simulink model "heart_model"  (R2015a)
settings: Solver=ode3  StartTime=0.0  StopTime=size(sasignal,1)  FixedStep=1  RelTol=1e-6  AbsTol=1e-6
values from neighbouring files (symbols this model uses):
  beta1 = [-1 -0.3 -0.09 -0.3 -0.3 -0.3 -0.3 -0.3 -0.3 -0.3 -0.3 -0.3 ... (33 elements, 1x33)]    [pacemaker_heart_params.mat]
  beta3 = [200 200 200 200 200 200 200 200 200 200 200 200 ... (33 elements, 1x33)]    [pacemaker_heart_params.mat]
  beta4 = [-0.05 -0.05 -0.02 -0.02 -0.02 -0.02 -0.02 -0.02 -0.02 -0.02 -0.02 -0.02 ... (33 elements, 1x33)]    [pacemaker_heart_params.mat]
  delay = [15.5648 23.2106666667 5.18826666667 12.0149333333 12.8341333333 10.9226666667 18.5685333333 9.55733333333 12.8341333333 4.36906666667 5.46133333333 9.8304 ... (34 elements, 1x34)]    [pacemaker_heart_params.mat]
  gain = [0.1 0.1 0.1 0.1 0.07 0.1 0.1 0.1 0.1 0.1 0.1 0.1 ... (33 elements, 1x33)]    [pacemaker_heart_params.mat]
libraries: simulink x40, dspsrcs4 x1
(part 3 of 5)

== system heart_model/Heart Model/VENTRICLE/RBB (12)/Subsystem3 ==
  q : Inport
  vreset : Inport  Port=2
  reset : Inport  Port=3
  I_st : Inport  Port=4
  vno : Inport  Port=5
  vin : Inport  Port=6
  win : Inport  Port=7
  Constant1 : Constant  Value=0
  Constant2 : Constant  Value=1/6
  Constant3 : Constant
  Gain1 : Gain  Gain=13
  IC : InitialCondition  Value=0
  Integrator : Integrator  ExternalReset=either  InitialConditionSource=external  LimitOutput=on  UpperSaturationLimit=138  ShowStatePort=on
  Math Function : Math  Operator=pow  SaturateOnIntegerOverflow=on
  Subsystem : Subsystem
  Subsystem2 : Subsystem
  Sum : Sum  Inputs=|++
  Switch : Switch  Threshold=0.1
  v : Outport
  vnext : Outport  Port=2
  wires:
  win/1 -> Subsystem/5(win)
  vin/1 -> Subsystem/4(vin), Subsystem2/4(vin)
  Integrator/State -> vnext/1
  Constant1/1 -> Switch/3
  vno/1 -> Switch/1, Switch/2
  Sum/1 -> Subsystem/3(f(vno))
  Switch/1 -> Math Function/1
  Constant3/1 -> Sum/2
  Gain1/1 -> Sum/1
  Math Function/1 -> Gain1/1
  Constant2/1 -> Math Function/2
  I_st/1 -> Subsystem2/1(I_st)
  reset/1 -> Integrator/2
  vreset/1 -> IC/1
  Subsystem2/1(vint) -> Integrator/1
  Subsystem/1(vgain) -> Subsystem2/3(vgain)
  Integrator/1 -> Subsystem/2(v), v/1
  IC/1 -> Integrator/3
  q/1 -> Subsystem/1(q), Subsystem2/2(q)

== system heart_model/Heart Model/VENTRICLE/RBB_m (11)/Subsystem3 ==
  q : Inport
  vreset : Inport  Port=2
  reset : Inport  Port=3
  I_st : Inport  Port=4
  vno : Inport  Port=5
  vin : Inport  Port=6
  win : Inport  Port=7
  Constant1 : Constant  Value=0
  Constant2 : Constant  Value=1/6
  Constant3 : Constant
  Gain1 : Gain  Gain=13
  IC : InitialCondition  Value=0
  Integrator : Integrator  ExternalReset=either  InitialConditionSource=external  LimitOutput=on  UpperSaturationLimit=138  ShowStatePort=on
  Math Function : Math  Operator=pow  SaturateOnIntegerOverflow=on
  Subsystem : Subsystem
  Subsystem2 : Subsystem
  Sum : Sum  Inputs=|++
  Switch : Switch  Threshold=0.1
  v : Outport
  vnext : Outport  Port=2
  wires:
  win/1 -> Subsystem/5(win)
  vin/1 -> Subsystem/4(vin), Subsystem2/4(vin)
  Integrator/State -> vnext/1
  Constant1/1 -> Switch/3
  vno/1 -> Switch/1, Switch/2
  Sum/1 -> Subsystem/3(f(vno))
  Switch/1 -> Math Function/1
  Constant3/1 -> Sum/2
  Gain1/1 -> Sum/1
  Math Function/1 -> Gain1/1
  Constant2/1 -> Math Function/2
  I_st/1 -> Subsystem2/1(I_st)
  reset/1 -> Integrator/2
  vreset/1 -> IC/1
  Subsystem2/1(vint) -> Integrator/1
  Subsystem/1(vgain) -> Subsystem2/3(vgain)
  Integrator/1 -> Subsystem/2(v), v/1
  IC/1 -> Integrator/3
  q/1 -> Subsystem/1(q), Subsystem2/2(q)

== system heart_model/Heart Model/VENTRICLE/RV (18)/Subsystem3 ==
  q : Inport
  vreset : Inport  Port=2
  reset : Inport  Port=3
  I_st : Inport  Port=4
  vno : Inport  Port=5
  vin : Inport  Port=6
  win : Inport  Port=7
  Constant1 : Constant  Value=0
  Constant2 : Constant  Value=1/6
  Constant3 : Constant
  Gain1 : Gain  Gain=13
  IC : InitialCondition  Value=0
  Integrator : Integrator  ExternalReset=either  InitialConditionSource=external  LimitOutput=on  UpperSaturationLimit=138  ShowStatePort=on
  Math Function : Math  Operator=pow  SaturateOnIntegerOverflow=on
  Subsystem : Subsystem
  Subsystem2 : Subsystem
  Sum : Sum  Inputs=|++
  Switch : Switch  Threshold=0.1
  v : Outport
  vnext : Outport  Port=2
  wires:
  win/1 -> Subsystem/5(win)
  vin/1 -> Subsystem/4(vin), Subsystem2/4(vin)
  Integrator/State -> vnext/1
  Constant1/1 -> Switch/3
  vno/1 -> Switch/1, Switch/2
  Sum/1 -> Subsystem/3(f(vno))
  Switch/1 -> Math Function/1
  Constant3/1 -> Sum/2
  Gain1/1 -> Sum/1
  Math Function/1 -> Gain1/1
  Constant2/1 -> Math Function/2
  I_st/1 -> Subsystem2/1(I_st)
  reset/1 -> Integrator/2
  vreset/1 -> IC/1
  Subsystem2/1(vint) -> Integrator/1
  Subsystem/1(vgain) -> Subsystem2/3(vgain)
  Integrator/1 -> Subsystem/2(v), v/1
  IC/1 -> Integrator/3
  q/1 -> Subsystem/1(q), Subsystem2/2(q)

== system heart_model/Heart Model/VENTRICLE/RVA (15)/Subsystem3 ==
  q : Inport
  vreset : Inport  Port=2
  reset : Inport  Port=3
  I_st : Inport  Port=4
  vno : Inport  Port=5
  vin : Inport  Port=6
  win : Inport  Port=7
  Constant1 : Constant  Value=0
  Constant2 : Constant  Value=1/6
  Constant3 : Constant
  Gain1 : Gain  Gain=13
  IC : InitialCondition  Value=0
  Integrator : Integrator  ExternalReset=either  InitialConditionSource=external  LimitOutput=on  UpperSaturationLimit=138  ShowStatePort=on
  Math Function : Math  Operator=pow  SaturateOnIntegerOverflow=on
  Subsystem : Subsystem
  Subsystem2 : Subsystem
  Sum : Sum  Inputs=|++
  Switch : Switch  Threshold=0.1
  v : Outport
  vnext : Outport  Port=2
  wires:
  win/1 -> Subsystem/5(win)
  vin/1 -> Subsystem/4(vin), Subsystem2/4(vin)
  Integrator/State -> vnext/1
  Constant1/1 -> Switch/3
  vno/1 -> Switch/1, Switch/2
  Sum/1 -> Subsystem/3(f(vno))
  Switch/1 -> Math Function/1
  Constant3/1 -> Sum/2
  Gain1/1 -> Sum/1
  Math Function/1 -> Gain1/1
  Constant2/1 -> Math Function/2
  I_st/1 -> Subsystem2/1(I_st)
  reset/1 -> Integrator/2
  vreset/1 -> IC/1
  Subsystem2/1(vint) -> Integrator/1
  Subsystem/1(vgain) -> Subsystem2/3(vgain)
  Integrator/1 -> Subsystem/2(v), v/1
  IC/1 -> Integrator/3
  q/1 -> Subsystem/1(q), Subsystem2/2(q)

== system heart_model/Heart Model/VENTRICLE/RV_m (17)/Subsystem3 ==
  q : Inport
  vreset : Inport  Port=2
  reset : Inport  Port=3
  I_st : Inport  Port=4
  vno : Inport  Port=5
  vin : Inport  Port=6
  win : Inport  Port=7
  Constant1 : Constant  Value=0
  Constant2 : Constant  Value=1/6
  Constant3 : Constant
  Gain1 : Gain  Gain=13
  IC : InitialCondition  Value=0
  Integrator : Integrator  ExternalReset=either  InitialConditionSource=external  LimitOutput=on  UpperSaturationLimit=138  ShowStatePort=on
  Math Function : Math  Operator=pow  SaturateOnIntegerOverflow=on
  Subsystem : Subsystem
  Subsystem2 : Subsystem
  Sum : Sum  Inputs=|++
  Switch : Switch  Threshold=0.1
  v : Outport
  vnext : Outport  Port=2
  wires:
  win/1 -> Subsystem/5(win)
  vin/1 -> Subsystem/4(vin), Subsystem2/4(vin)
  Integrator/State -> vnext/1
  Constant1/1 -> Switch/3
  vno/1 -> Switch/1, Switch/2
  Sum/1 -> Subsystem/3(f(vno))
  Switch/1 -> Math Function/1
  Constant3/1 -> Sum/2
  Gain1/1 -> Sum/1
  Math Function/1 -> Gain1/1
  Constant2/1 -> Math Function/2
  I_st/1 -> Subsystem2/1(I_st)
  reset/1 -> Integrator/2
  vreset/1 -> IC/1
  Subsystem2/1(vint) -> Integrator/1
  Subsystem/1(vgain) -> Subsystem2/3(vgain)
  Integrator/1 -> Subsystem/2(v), v/1
  IC/1 -> Integrator/3
  q/1 -> Subsystem/1(q), Subsystem2/2(q)

== system heart_model/Heart Model/VENTRICLE/SEP_LV (27)/Subsystem3 ==
  q : Inport
  vreset : Inport  Port=2
  reset : Inport  Port=3
  I_st : Inport  Port=4
  vno : Inport  Port=5
  vin : Inport  Port=6
  win : Inport  Port=7
  Constant1 : Constant  Value=0
  Constant2 : Constant  Value=1/6
  Constant3 : Constant
  Gain1 : Gain  Gain=13
  IC : InitialCondition  Value=0
  Integrator : Integrator  ExternalReset=either  InitialConditionSource=external  LimitOutput=on  UpperSaturationLimit=138  ShowStatePort=on
  Math Function : Math  Operator=pow  SaturateOnIntegerOverflow=on
  Subsystem : Subsystem
  Subsystem2 : Subsystem
  Sum : Sum  Inputs=|++
  Switch : Switch  Threshold=0.1
  v : Outport
  vnext : Outport  Port=2
  wires:
  win/1 -> Subsystem/5(win)
  vin/1 -> Subsystem/4(vin), Subsystem2/4(vin)
  Integrator/State -> vnext/1
  Constant1/1 -> Switch/3
  vno/1 -> Switch/1, Switch/2
  Sum/1 -> Subsystem/3(f(vno))
  Switch/1 -> Math Function/1
  Constant3/1 -> Sum/2
  Gain1/1 -> Sum/1
  Math Function/1 -> Gain1/1
  Constant2/1 -> Math Function/2
  I_st/1 -> Subsystem2/1(I_st)
  reset/1 -> Integrator/2
  vreset/1 -> IC/1
  Subsystem2/1(vint) -> Integrator/1
  Subsystem/1(vgain) -> Subsystem2/3(vgain)
  Integrator/1 -> Subsystem/2(v), v/1
  IC/1 -> Integrator/3
  q/1 -> Subsystem/1(q), Subsystem2/2(q)

== system heart_model/Heart Model/VENTRICLE/SEP_LV_m (26)/Subsystem3 ==
  q : Inport
  vreset : Inport  Port=2
  reset : Inport  Port=3
  I_st : Inport  Port=4
  vno : Inport  Port=5
  vin : Inport  Port=6
  win : Inport  Port=7
  Constant1 : Constant  Value=0
  Constant2 : Constant  Value=1/6
  Constant3 : Constant
  Gain1 : Gain  Gain=13
  IC : InitialCondition  Value=0
  Integrator : Integrator  ExternalReset=either  InitialConditionSource=external  LimitOutput=on  UpperSaturationLimit=138  ShowStatePort=on
  Math Function : Math  Operator=pow  SaturateOnIntegerOverflow=on
  Subsystem : Subsystem
  Subsystem2 : Subsystem
  Sum : Sum  Inputs=|++
  Switch : Switch  Threshold=0.1
  v : Outport
  vnext : Outport  Port=2
  wires:
  win/1 -> Subsystem/5(win)
  vin/1 -> Subsystem/4(vin), Subsystem2/4(vin)
  Integrator/State -> vnext/1
  Constant1/1 -> Switch/3
  vno/1 -> Switch/1, Switch/2
  Sum/1 -> Subsystem/3(f(vno))
  Switch/1 -> Math Function/1
  Constant3/1 -> Sum/2
  Gain1/1 -> Sum/1
  Math Function/1 -> Gain1/1
  Constant2/1 -> Math Function/2
  I_st/1 -> Subsystem2/1(I_st)
  reset/1 -> Integrator/2
  vreset/1 -> IC/1
  Subsystem2/1(vint) -> Integrator/1
  Subsystem/1(vgain) -> Subsystem2/3(vgain)
  Integrator/1 -> Subsystem/2(v), v/1
  IC/1 -> Integrator/3
  q/1 -> Subsystem/1(q), Subsystem2/2(q)

== system heart_model/Heart Model/VENTRICLE/SEP_RV (25)/Subsystem3 ==
  q : Inport
  vreset : Inport  Port=2
  reset : Inport  Port=3
  I_st : Inport  Port=4
  vno : Inport  Port=5
  vin : Inport  Port=6
  win : Inport  Port=7
  Constant1 : Constant  Value=0
  Constant2 : Constant  Value=1/6
  Constant3 : Constant
  Gain1 : Gain  Gain=13
  IC : InitialCondition  Value=0
  Integrator : Integrator  ExternalReset=either  InitialConditionSource=external  LimitOutput=on  UpperSaturationLimit=138  ShowStatePort=on
  Math Function : Math  Operator=pow  SaturateOnIntegerOverflow=on
  Subsystem : Subsystem
  Subsystem2 : Subsystem
  Sum : Sum  Inputs=|++
  Switch : Switch  Threshold=0.1
  v : Outport
  vnext : Outport  Port=2
  wires:
  win/1 -> Subsystem/5(win)
  vin/1 -> Subsystem/4(vin), Subsystem2/4(vin)
  Integrator/State -> vnext/1
  Constant1/1 -> Switch/3
  vno/1 -> Switch/1, Switch/2
  Sum/1 -> Subsystem/3(f(vno))
  Switch/1 -> Math Function/1
  Constant3/1 -> Sum/2
  Gain1/1 -> Sum/1
  Math Function/1 -> Gain1/1
  Constant2/1 -> Math Function/2
  I_st/1 -> Subsystem2/1(I_st)
  reset/1 -> Integrator/2
  vreset/1 -> IC/1
  Subsystem2/1(vint) -> Integrator/1
  Subsystem/1(vgain) -> Subsystem2/3(vgain)
  Integrator/1 -> Subsystem/2(v), v/1
  IC/1 -> Integrator/3
  q/1 -> Subsystem/1(q), Subsystem2/2(q)

== system heart_model/Heart Model/VENTRICLE/SEP_RV_m (24)/Subsystem3 ==
  q : Inport
  vreset : Inport  Port=2
  reset : Inport  Port=3
  I_st : Inport  Port=4
  vno : Inport  Port=5
  vin : Inport  Port=6
  win : Inport  Port=7
  Constant1 : Constant  Value=0
  Constant2 : Constant  Value=1/6
  Constant3 : Constant
  Gain1 : Gain  Gain=13
  IC : InitialCondition  Value=0
  Integrator : Integrator  ExternalReset=either  InitialConditionSource=external  LimitOutput=on  UpperSaturationLimit=138  ShowStatePort=on
  Math Function : Math  Operator=pow  SaturateOnIntegerOverflow=on
  Subsystem : Subsystem
  Subsystem2 : Subsystem
  Sum : Sum  Inputs=|++
  Switch : Switch  Threshold=0.1
  v : Outport
  vnext : Outport  Port=2
  wires:
  win/1 -> Subsystem/5(win)
  vin/1 -> Subsystem/4(vin), Subsystem2/4(vin)
  Integrator/State -> vnext/1
  Constant1/1 -> Switch/3
  vno/1 -> Switch/1, Switch/2
  Sum/1 -> Subsystem/3(f(vno))
  Switch/1 -> Math Function/1
  Constant3/1 -> Sum/2
  Gain1/1 -> Sum/1
  Math Function/1 -> Gain1/1
  Constant2/1 -> Math Function/2
  I_st/1 -> Subsystem2/1(I_st)
  reset/1 -> Integrator/2
  vreset/1 -> IC/1
  Subsystem2/1(vint) -> Integrator/1
  Subsystem/1(vgain) -> Subsystem2/3(vgain)
  Integrator/1 -> Subsystem/2(v), v/1
  IC/1 -> Integrator/3
  q/1 -> Subsystem/1(q), Subsystem2/2(q)

== system heart_model/Heart Model/ATRIUM/Bach (8)/Subsystem3/Subsystem ==
  q : Inport
  v : Inport  Port=2
  f(vno) : Inport  Port=3
  vin : Inport  Port=4
  win : Inport  Port=5
  Gain3 : Gain  Gain=-1
  Multiport Switch : MultiPortSwitch  Inputs=4
  Product : Product  RndMeth=Zero
  Product1 : Product  RndMeth=Zero
  Sum : Sum  Inputs=|++
  Sum1 : Sum  Inputs=|++
  beta1 : Gain  Gain=beta1(8)
  beta3 : Gain  Gain=beta3(8)
  beta4 : Gain  Gain=beta4(8)
  vgain : Outport
  wires:
  Gain3/1 -> Product1/2
  Product1/1 -> Multiport Switch/3, Sum1/2
  Sum1/1 -> Multiport Switch/2
  Sum/1 -> Sum1/1
  win/1 -> Gain3/1
  vin/1 -> Sum/1
  beta1/1 -> Sum/2
  f(vno)/1 -> Product/2
  beta4/1 -> Product/1
  Product/1 -> Multiport Switch/5
  v/1 -> Product1/1, beta4/1, beta3/1, beta1/1
  beta3/1 -> Multiport Switch/4
  Multiport Switch/1 -> vgain/1
  q/1 -> Multiport Switch/1

== system heart_model/Heart Model/ATRIUM/Bach (8)/Subsystem3/Subsystem2 ==
  I_st : Inport
  q : Inport  Port=2
  vgain : Inport  Port=3
  vin : Inport  Port=4
  Compare To Constant : simulink/Logic and Bit Operations/Compare To Constant  relop===  const=2  OutDataTypeStr=uint8
  Sum : Sum  Inputs=|++
  Sum1 : Sum  Inputs=|++
  Switch : Switch  Criteria=u2 ~= 0
  vint : Outport
  wires:
  Sum1/1 -> Switch/1
  Sum/1 -> Sum1/2
  vin/1 -> Sum/2
  I_st/1 -> Sum/1
  vgain/1 -> Sum1/1, Switch/3
  Switch/1 -> vint/1
  q/1 -> Compare To Constant/1
  Compare To Constant/1 -> Switch/2

== system heart_model/Heart Model/ATRIUM/CS_LA (29)/Subsystem3/Subsystem ==
  q : Inport
  v : Inport  Port=2
  f(vno) : Inport  Port=3
  vin : Inport  Port=4
  win : Inport  Port=5
  Gain3 : Gain  Gain=-1
  Multiport Switch : MultiPortSwitch  Inputs=4
  Product : Product  RndMeth=Zero
  Product1 : Product  RndMeth=Zero
  Sum : Sum  Inputs=|++
  Sum1 : Sum  Inputs=|++
  beta1 : Gain  Gain=beta1(29)
  beta3 : Gain  Gain=beta3(29)
  beta4 : Gain  Gain=beta4(29)
  vgain : Outport
  wires:
  Gain3/1 -> Product1/2
  Product1/1 -> Multiport Switch/3, Sum1/2
  Sum1/1 -> Multiport Switch/2
  Sum/1 -> Sum1/1
  win/1 -> Gain3/1
  vin/1 -> Sum/1
  beta1/1 -> Sum/2
  f(vno)/1 -> Product/2
  beta4/1 -> Product/1
  Product/1 -> Multiport Switch/5
  v/1 -> Product1/1, beta4/1, beta3/1, beta1/1
  beta3/1 -> Multiport Switch/4
  Multiport Switch/1 -> vgain/1
  q/1 -> Multiport Switch/1

== system heart_model/Heart Model/ATRIUM/CS_LA (29)/Subsystem3/Subsystem2 ==
  I_st : Inport
  q : Inport  Port=2
  vgain : Inport  Port=3
  vin : Inport  Port=4
  Compare To Constant : simulink/Logic and Bit Operations/Compare To Constant  relop===  const=2  OutDataTypeStr=uint8
  Sum : Sum  Inputs=|++
  Sum1 : Sum  Inputs=|++
  Switch : Switch  Criteria=u2 ~= 0
  vint : Outport
  wires:
  Sum1/1 -> Switch/1
  Sum/1 -> Sum1/2
  vin/1 -> Sum/2
  I_st/1 -> Sum/1
  vgain/1 -> Sum1/1, Switch/3
  Switch/1 -> vint/1
  q/1 -> Compare To Constant/1
  Compare To Constant/1 -> Switch/2

== system heart_model/Heart Model/ATRIUM/CT (2)/Subsystem3/Subsystem ==
  q : Inport
  v : Inport  Port=2
  f(vno) : Inport  Port=3
  vin : Inport  Port=4
  win : Inport  Port=5
  Gain3 : Gain  Gain=-1
  Multiport Switch : MultiPortSwitch  Inputs=4
  Product : Product  RndMeth=Zero
  Product1 : Product  RndMeth=Zero
  Sum : Sum  Inputs=|++
  Sum1 : Sum  Inputs=|++
  beta1 : Gain  Gain=beta1(2)
  beta3 : Gain  Gain=beta3(2)
  beta4 : Gain  Gain=beta4(2)
  vgain : Outport
  wires:
  Gain3/1 -> Product1/2
  Product1/1 -> Multiport Switch/3, Sum1/2
  Sum1/1 -> Multiport Switch/2
  Sum/1 -> Sum1/1
  win/1 -> Gain3/1
  vin/1 -> Sum/1
  beta1/1 -> Sum/2
  f(vno)/1 -> Product/2
  beta4/1 -> Product/1
  Product/1 -> Multiport Switch/5
  v/1 -> Product1/1, beta4/1, beta3/1, beta1/1
  beta3/1 -> Multiport Switch/4
  Multiport Switch/1 -> vgain/1
  q/1 -> Multiport Switch/1

== system heart_model/Heart Model/ATRIUM/CT (2)/Subsystem3/Subsystem2 ==
  I_st : Inport
  q : Inport  Port=2
  vgain : Inport  Port=3
  vin : Inport  Port=4
  Compare To Constant : simulink/Logic and Bit Operations/Compare To Constant  relop===  const=2  OutDataTypeStr=uint8
  Sum : Sum  Inputs=|++
  Sum1 : Sum  Inputs=|++
  Switch : Switch  Criteria=u2 ~= 0
  vint : Outport
  wires:
  Sum1/1 -> Switch/1
  Sum/1 -> Sum1/2
  vin/1 -> Sum/2
  I_st/1 -> Sum/1
  vgain/1 -> Sum1/1, Switch/3
  Switch/1 -> vint/1
  q/1 -> Compare To Constant/1
  Compare To Constant/1 -> Switch/2

== system heart_model/Heart Model/ATRIUM/CT_a (21)/Subsystem3/Subsystem ==
  q : Inport
  v : Inport  Port=2
  f(vno) : Inport  Port=3
  vin : Inport  Port=4
  win : Inport  Port=5
  Gain3 : Gain  Gain=-1
  Multiport Switch : MultiPortSwitch  Inputs=4
  Product : Product  RndMeth=Zero
  Product1 : Product  RndMeth=Zero
  Sum : Sum  Inputs=|++
  Sum1 : Sum  Inputs=|++
  beta1 : Gain  Gain=beta1(21)
  beta3 : Gain  Gain=beta3(21)
  beta4 : Gain  Gain=beta4(21)
  vgain : Outport
  wires:
  Gain3/1 -> Product1/2
  Product1/1 -> Multiport Switch/3, Sum1/2
  Sum1/1 -> Multiport Switch/2
  Sum/1 -> Sum1/1
  win/1 -> Gain3/1
  vin/1 -> Sum/1
  beta1/1 -> Sum/2
  f(vno)/1 -> Product/2
  beta4/1 -> Product/1
  Product/1 -> Multiport Switch/5
  v/1 -> Product1/1, beta4/1, beta3/1, beta1/1
  beta3/1 -> Multiport Switch/4
  Multiport Switch/1 -> vgain/1
  q/1 -> Multiport Switch/1

== system heart_model/Heart Model/ATRIUM/CT_a (21)/Subsystem3/Subsystem2 ==
  I_st : Inport
  q : Inport  Port=2
  vgain : Inport  Port=3
  vin : Inport  Port=4
  Compare To Constant : simulink/Logic and Bit Operations/Compare To Constant  relop===  const=2  OutDataTypeStr=uint8
  Sum : Sum  Inputs=|++
  Sum1 : Sum  Inputs=|++
  Switch : Switch  Criteria=u2 ~= 0
  vint : Outport
  wires:
  Sum1/1 -> Switch/1
  Sum/1 -> Sum1/2
  vin/1 -> Sum/2
  I_st/1 -> Sum/1
  vgain/1 -> Sum1/1, Switch/3
  Switch/1 -> vint/1
  q/1 -> Compare To Constant/1
  Compare To Constant/1 -> Switch/2

== system heart_model/Heart Model/ATRIUM/Fast (32)/Subsystem3/Subsystem ==
  q : Inport
  v : Inport  Port=2
  f(vno) : Inport  Port=3
  vin : Inport  Port=4
  win : Inport  Port=5
  Gain3 : Gain  Gain=-1
  Multiport Switch : MultiPortSwitch  Inputs=4
  Product : Product  RndMeth=Zero
  Product1 : Product  RndMeth=Zero
  Sum : Sum  Inputs=|++
  Sum1 : Sum  Inputs=|++
  beta1 : Gain  Gain=beta1(32)
  beta3 : Gain  Gain=beta3(32)
  beta4 : Gain  Gain=beta4(32)
  vgain : Outport
  wires:
  Gain3/1 -> Product1/2
  Product1/1 -> Multiport Switch/3, Sum1/2
  Sum1/1 -> Multiport Switch/2
  Sum/1 -> Sum1/1
  win/1 -> Gain3/1
  vin/1 -> Sum/1
  beta1/1 -> Sum/2
  f(vno)/1 -> Product/2
  beta4/1 -> Product/1
  Product/1 -> Multiport Switch/5
  v/1 -> Product1/1, beta4/1, beta3/1, beta1/1
  beta3/1 -> Multiport Switch/4
  Multiport Switch/1 -> vgain/1
  q/1 -> Multiport Switch/1

== system heart_model/Heart Model/ATRIUM/Fast (32)/Subsystem3/Subsystem2 ==
  I_st : Inport
  q : Inport  Port=2
  vgain : Inport  Port=3
  vin : Inport  Port=4
  Compare To Constant : simulink/Logic and Bit Operations/Compare To Constant  relop===  const=2  OutDataTypeStr=uint8
  Sum : Sum  Inputs=|++
  Sum1 : Sum  Inputs=|++
  Switch : Switch  Criteria=u2 ~= 0
  vint : Outport
  wires:
  Sum1/1 -> Switch/1
  Sum/1 -> Sum1/2
  vin/1 -> Sum/2
  I_st/1 -> Sum/1
  vgain/1 -> Sum1/1, Switch/3
  Switch/1 -> vint/1
  q/1 -> Compare To Constant/1
  Compare To Constant/1 -> Switch/2

== system heart_model/Heart Model/ATRIUM/Fast_b (33)/Subsystem3/Subsystem ==
  q : Inport
  v : Inport  Port=2
  f(vno) : Inport  Port=3
  vin : Inport  Port=4
  win : Inport  Port=5
  Gain3 : Gain  Gain=-1
  Multiport Switch : MultiPortSwitch  Inputs=4
  Product : Product  RndMeth=Zero
  Product1 : Product  RndMeth=Zero
  Sum : Sum  Inputs=|++
  Sum1 : Sum  Inputs=|++
  beta1 : Gain  Gain=beta1(33)
  beta3 : Gain  Gain=beta3(33)
  beta4 : Gain  Gain=beta4(33)
  vgain : Outport
  wires:
  Gain3/1 -> Product1/2
  Product1/1 -> Multiport Switch/3, Sum1/2
  Sum1/1 -> Multiport Switch/2
  Sum/1 -> Sum1/1
  win/1 -> Gain3/1
  vin/1 -> Sum/1
  beta1/1 -> Sum/2
  f(vno)/1 -> Product/2
  beta4/1 -> Product/1
  Product/1 -> Multiport Switch/5
  v/1 -> Product1/1, beta4/1, beta3/1, beta1/1
  beta3/1 -> Multiport Switch/4
  Multiport Switch/1 -> vgain/1
  q/1 -> Multiport Switch/1

== system heart_model/Heart Model/ATRIUM/Fast_b (33)/Subsystem3/Subsystem2 ==
  I_st : Inport
  q : Inport  Port=2
  vgain : Inport  Port=3
  vin : Inport  Port=4
  Compare To Constant : simulink/Logic and Bit Operations/Compare To Constant  relop===  const=2  OutDataTypeStr=uint8
  Sum : Sum  Inputs=|++
  Sum1 : Sum  Inputs=|++
  Switch : Switch  Criteria=u2 ~= 0
  vint : Outport
  wires:
  Sum1/1 -> Switch/1
  Sum/1 -> Sum1/2
  vin/1 -> Sum/2
  I_st/1 -> Sum/1
  vgain/1 -> Sum1/1, Switch/3
  Switch/1 -> vint/1
  q/1 -> Compare To Constant/1
  Compare To Constant/1 -> Switch/2

== system heart_model/Heart Model/ATRIUM/LA (10)/Subsystem3/Subsystem ==
  q : Inport
  v : Inport  Port=2
  f(vno) : Inport  Port=3
  vin : Inport  Port=4
  win : Inport  Port=5
  Gain3 : Gain  Gain=-1
  Multiport Switch : MultiPortSwitch  Inputs=4
  Product : Product  RndMeth=Zero
  Product1 : Product  RndMeth=Zero
  Sum : Sum  Inputs=|++
  Sum1 : Sum  Inputs=|++
  beta1 : Gain  Gain=beta1(10)
  beta3 : Gain  Gain=beta3(10)
  beta4 : Gain  Gain=beta4(10)
  vgain : Outport
  wires:
  Gain3/1 -> Product1/2
  Product1/1 -> Multiport Switch/3, Sum1/2
  Sum1/1 -> Multiport Switch/2
  Sum/1 -> Sum1/1
  win/1 -> Gain3/1
  vin/1 -> Sum/1
  beta1/1 -> Sum/2
  f(vno)/1 -> Product/2
  beta4/1 -> Product/1
  Product/1 -> Multiport Switch/5
  v/1 -> Product1/1, beta4/1, beta3/1, beta1/1
  beta3/1 -> Multiport Switch/4
  Multiport Switch/1 -> vgain/1
  q/1 -> Multiport Switch/1

== system heart_model/Heart Model/ATRIUM/LA (10)/Subsystem3/Subsystem2 ==
  I_st : Inport
  q : Inport  Port=2
  vgain : Inport  Port=3
  vin : Inport  Port=4
  Compare To Constant : simulink/Logic and Bit Operations/Compare To Constant  relop===  const=2  OutDataTypeStr=uint8
  Sum : Sum  Inputs=|++
  Sum1 : Sum  Inputs=|++
  Switch : Switch  Criteria=u2 ~= 0
  vint : Outport
  wires:
  Sum1/1 -> Switch/1
  Sum/1 -> Sum1/2
  vin/1 -> Sum/2
  I_st/1 -> Sum/1
  vgain/1 -> Sum1/1, Switch/3
  Switch/1 -> vint/1
  q/1 -> Compare To Constant/1
  Compare To Constant/1 -> Switch/2

== system heart_model/Heart Model/ATRIUM/LA_a (9)/Subsystem3/Subsystem ==
  q : Inport
  v : Inport  Port=2
  f(vno) : Inport  Port=3
  vin : Inport  Port=4
  win : Inport  Port=5
  Gain3 : Gain  Gain=-1
  Multiport Switch : MultiPortSwitch  Inputs=4
  Product : Product  RndMeth=Zero
  Product1 : Product  RndMeth=Zero
  Sum : Sum  Inputs=|++
  Sum1 : Sum  Inputs=|++
  beta1 : Gain  Gain=beta1(9)
  beta3 : Gain  Gain=beta3(9)
  beta4 : Gain  Gain=beta4(9)
  vgain : Outport
  wires:
  Gain3/1 -> Product1/2
  Product1/1 -> Multiport Switch/3, Sum1/2
  Sum1/1 -> Multiport Switch/2
  Sum/1 -> Sum1/1
  win/1 -> Gain3/1
  vin/1 -> Sum/1
  beta1/1 -> Sum/2
  f(vno)/1 -> Product/2
  beta4/1 -> Product/1
  Product/1 -> Multiport Switch/5
  v/1 -> Product1/1, beta4/1, beta3/1, beta1/1
  beta3/1 -> Multiport Switch/4
  Multiport Switch/1 -> vgain/1
  q/1 -> Multiport Switch/1

== system heart_model/Heart Model/ATRIUM/LA_a (9)/Subsystem3/Subsystem2 ==
  I_st : Inport
  q : Inport  Port=2
  vgain : Inport  Port=3
  vin : Inport  Port=4
  Compare To Constant : simulink/Logic and Bit Operations/Compare To Constant  relop===  const=2  OutDataTypeStr=uint8
  Sum : Sum  Inputs=|++
  Sum1 : Sum  Inputs=|++
  Switch : Switch  Criteria=u2 ~= 0
  vint : Outport
  wires:
  Sum1/1 -> Switch/1
  Sum/1 -> Sum1/2
  vin/1 -> Sum/2
  I_st/1 -> Sum/1
  vgain/1 -> Sum1/1, Switch/3
  Switch/1 -> vint/1
  q/1 -> Compare To Constant/1
  Compare To Constant/1 -> Switch/2

== system heart_model/Heart Model/ATRIUM/OS (4)/Subsystem3/Subsystem ==
  q : Inport
  v : Inport  Port=2
  f(vno) : Inport  Port=3
  vin : Inport  Port=4
  win : Inport  Port=5
  Gain3 : Gain  Gain=-1
  Multiport Switch : MultiPortSwitch  Inputs=4
  Product : Product  RndMeth=Zero
  Product1 : Product  RndMeth=Zero
  Sum : Sum  Inputs=|++
  Sum1 : Sum  Inputs=|++
  beta1 : Gain  Gain=beta1(4)
  beta3 : Gain  Gain=beta3(4)
  beta4 : Gain  Gain=beta4(4)
  vgain : Outport
  wires:
  Gain3/1 -> Product1/2
  Product1/1 -> Multiport Switch/3, Sum1/2
  Sum1/1 -> Multiport Switch/2
  Sum/1 -> Sum1/1
  win/1 -> Gain3/1
  vin/1 -> Sum/1
  beta1/1 -> Sum/2
  f(vno)/1 -> Product/2
  beta4/1 -> Product/1
  Product/1 -> Multiport Switch/5
  v/1 -> Product1/1, beta4/1, beta3/1, beta1/1
  beta3/1 -> Multiport Switch/4
  Multiport Switch/1 -> vgain/1
  q/1 -> Multiport Switch/1

== system heart_model/Heart Model/ATRIUM/OS (4)/Subsystem3/Subsystem2 ==
  I_st : Inport
  q : Inport  Port=2
  vgain : Inport  Port=3
  Compare To Constant : simulink/Logic and Bit Operations/Compare To Constant  relop===  const=2  OutDataTypeStr=uint8
  Switch : Switch  Criteria=u2 ~= 0
  vint : Outport
  wires:
  I_st/1 -> Switch/1
  vgain/1 -> Switch/3
  Switch/1 -> vint/1
  q/1 -> Compare To Constant/1
  Compare To Constant/1 -> Switch/2

== system heart_model/Heart Model/ATRIUM/RA (23)/Subsystem3/Subsystem ==
  q : Inport
  v : Inport  Port=2
  f(vno) : Inport  Port=3
  vin : Inport  Port=4
  win : Inport  Port=5
  Gain3 : Gain  Gain=-1
  Multiport Switch : MultiPortSwitch  Inputs=4
  Product : Product  RndMeth=Zero
  Product1 : Product  RndMeth=Zero
  Sum : Sum  Inputs=|++
  Sum1 : Sum  Inputs=|++
  beta1 : Gain  Gain=beta1(23)
  beta3 : Gain  Gain=beta3(23)
  beta4 : Gain  Gain=beta4(23)
  vgain : Outport
  wires:
  Gain3/1 -> Product1/2
  Product1/1 -> Multiport Switch/3, Sum1/2
  Sum1/1 -> Multiport Switch/2
  Sum/1 -> Sum1/1
  win/1 -> Gain3/1
  vin/1 -> Sum/1
  beta1/1 -> Sum/2
  f(vno)/1 -> Product/2
  beta4/1 -> Product/1
  Product/1 -> Multiport Switch/5
  v/1 -> Product1/1, beta4/1, beta3/1, beta1/1
  beta3/1 -> Multiport Switch/4
  Multiport Switch/1 -> vgain/1
  q/1 -> Multiport Switch/1

== system heart_model/Heart Model/ATRIUM/RA (23)/Subsystem3/Subsystem2 ==
  I_st : Inport
  q : Inport  Port=2
  vgain : Inport  Port=3
  vin : Inport  Port=4
  Compare To Constant : simulink/Logic and Bit Operations/Compare To Constant  relop===  const=2  OutDataTypeStr=uint8
  Sum : Sum  Inputs=|++
  Sum1 : Sum  Inputs=|++
  Switch : Switch  Criteria=u2 ~= 0
  vint : Outport
  wires:
  Sum1/1 -> Switch/1
  Sum/1 -> Sum1/2
  vin/1 -> Sum/2
  I_st/1 -> Sum/1
  vgain/1 -> Sum1/1, Switch/3
  Switch/1 -> vint/1
  q/1 -> Compare To Constant/1
  Compare To Constant/1 -> Switch/2

== system heart_model/Heart Model/ATRIUM/RA_a (22)/Subsystem3/Subsystem ==
  q : Inport
  v : Inport  Port=2
  f(vno) : Inport  Port=3
  vin : Inport  Port=4
  win : Inport  Port=5
  Gain3 : Gain  Gain=-1
  Multiport Switch : MultiPortSwitch  Inputs=4
  Product : Product  RndMeth=Zero
  Product1 : Product  RndMeth=Zero
  Sum : Sum  Inputs=|++
  Sum1 : Sum  Inputs=|++
  beta1 : Gain  Gain=beta1(22)
  beta3 : Gain  Gain=beta3(22)
  beta4 : Gain  Gain=beta4(22)
  vgain : Outport
  wires:
  Gain3/1 -> Product1/2
  Product1/1 -> Multiport Switch/3, Sum1/2
  Sum1/1 -> Multiport Switch/2
  Sum/1 -> Sum1/1
  win/1 -> Gain3/1
  vin/1 -> Sum/1
  beta1/1 -> Sum/2
  f(vno)/1 -> Product/2
  beta4/1 -> Product/1
  Product/1 -> Multiport Switch/5
  v/1 -> Product1/1, beta4/1, beta3/1, beta1/1
  beta3/1 -> Multiport Switch/4
  Multiport Switch/1 -> vgain/1
  q/1 -> Multiport Switch/1

== system heart_model/Heart Model/ATRIUM/RA_a (22)/Subsystem3/Subsystem2 ==
  I_st : Inport
  q : Inport  Port=2
  vgain : Inport  Port=3
  vin : Inport  Port=4
  Compare To Constant : simulink/Logic and Bit Operations/Compare To Constant  relop===  const=2  OutDataTypeStr=uint8
  Sum : Sum  Inputs=|++
  Sum1 : Sum  Inputs=|++
  Switch : Switch  Criteria=u2 ~= 0
  vint : Outport
  wires:
  Sum1/1 -> Switch/1
  Sum/1 -> Sum1/2
  vin/1 -> Sum/2
  I_st/1 -> Sum/1
  vgain/1 -> Sum1/1, Switch/3
  Switch/1 -> vint/1
  q/1 -> Compare To Constant/1
  Compare To Constant/1 -> Switch/2

== system heart_model/Heart Model/ATRIUM/Slow_a (31)/Subsystem3/Subsystem ==
  q : Inport
  v : Inport  Port=2
  f(vno) : Inport  Port=3
  vin : Inport  Port=4
  win : Inport  Port=5
  Gain3 : Gain  Gain=-1
  Multiport Switch : MultiPortSwitch  Inputs=4
  Product : Product  RndMeth=Zero
  Product1 : Product  RndMeth=Zero
  Sum : Sum  Inputs=|++
  Sum1 : Sum  Inputs=|++
  beta1 : Gain  Gain=beta1(31)
  beta3 : Gain  Gain=beta3(31)
  beta4 : Gain  Gain=beta4(31)
  vgain : Outport
  wires:
  Gain3/1 -> Product1/2
  Product1/1 -> Multiport Switch/3, Sum1/2
  Sum1/1 -> Multiport Switch/2
  Sum/1 -> Sum1/1
  win/1 -> Gain3/1
  vin/1 -> Sum/1
  beta1/1 -> Sum/2
  f(vno)/1 -> Product/2
  beta4/1 -> Product/1
  Product/1 -> Multiport Switch/5
  v/1 -> Product1/1, beta4/1, beta3/1, beta1/1
  beta3/1 -> Multiport Switch/4
  Multiport Switch/1 -> vgain/1
  q/1 -> Multiport Switch/1

== system heart_model/Heart Model/ATRIUM/Slow_a (31)/Subsystem3/Subsystem2 ==
  I_st : Inport
  q : Inport  Port=2
  vgain : Inport  Port=3
  vin : Inport  Port=4
  Compare To Constant : simulink/Logic and Bit Operations/Compare To Constant  relop===  const=2  OutDataTypeStr=uint8
  Sum : Sum  Inputs=|++
  Sum1 : Sum  Inputs=|++
  Switch : Switch  Criteria=u2 ~= 0
  vint : Outport
  wires:
  Sum1/1 -> Switch/1
  Sum/1 -> Sum1/2
  vin/1 -> Sum/2
  I_st/1 -> Sum/1
  vgain/1 -> Sum1/1, Switch/3
  Switch/1 -> vint/1
  q/1 -> Compare To Constant/1
  Compare To Constant/1 -> Switch/2

== system heart_model/Heart Model/ATRIUM/Slow_b (30)/Subsystem3/Subsystem ==
  q : Inport
  v : Inport  Port=2
  f(vno) : Inport  Port=3
  vin : Inport  Port=4
  win : Inport  Port=5
  Gain3 : Gain  Gain=-1
  Multiport Switch : MultiPortSwitch  Inputs=4
  Product : Product  RndMeth=Zero
  Product1 : Product  RndMeth=Zero
  Sum : Sum  Inputs=|++
  Sum1 : Sum  Inputs=|++
  beta1 : Gain  Gain=beta1(30)
  beta3 : Gain  Gain=beta3(30)
  beta4 : Gain  Gain=beta4(30)
  vgain : Outport
  wires:
  Gain3/1 -> Product1/2
  Product1/1 -> Multiport Switch/3, Sum1/2
  Sum1/1 -> Multiport Switch/2
  Sum/1 -> Sum1/1
  win/1 -> Gain3/1
  vin/1 -> Sum/1
  beta1/1 -> Sum/2
  f(vno)/1 -> Product/2
  beta4/1 -> Product/1
  Product/1 -> Multiport Switch/5
  v/1 -> Product1/1, beta4/1, beta3/1, beta1/1
  beta3/1 -> Multiport Switch/4
  Multiport Switch/1 -> vgain/1
  q/1 -> Multiport Switch/1

== system heart_model/Heart Model/ATRIUM/Slow_b (30)/Subsystem3/Subsystem2 ==
  I_st : Inport
  q : Inport  Port=2
  vgain : Inport  Port=3
  vin : Inport  Port=4
  Compare To Constant : simulink/Logic and Bit Operations/Compare To Constant  relop===  const=2  OutDataTypeStr=uint8
  Sum : Sum  Inputs=|++
  Sum1 : Sum  Inputs=|++
  Switch : Switch  Criteria=u2 ~= 0
  vint : Outport
  wires:
  Sum1/1 -> Switch/1
  Sum/1 -> Sum1/2
  vin/1 -> Sum/2
  I_st/1 -> Sum/1
  vgain/1 -> Sum1/1, Switch/3
  Switch/1 -> vint/1
  q/1 -> Compare To Constant/1
  Compare To Constant/1 -> Switch/2

== system heart_model/Heart Model/VENTRICLE/CS_LV (28)/Subsystem3/Subsystem ==
  q : Inport
  v : Inport  Port=2
  f(vno) : Inport  Port=3
  vin : Inport  Port=4
  win : Inport  Port=5
  Gain3 : Gain  Gain=-1
  Multiport Switch : MultiPortSwitch  Inputs=4
  Product : Product  RndMeth=Zero
  Product1 : Product  RndMeth=Zero
  Sum : Sum  Inputs=|++
  Sum1 : Sum  Inputs=|++
  beta1 : Gain  Gain=beta1(28)
  beta3 : Gain  Gain=beta3(28)
  beta4 : Gain  Gain=beta4(28)
  vgain : Outport
  wires:
  Gain3/1 -> Product1/2
  Product1/1 -> Multiport Switch/3, Sum1/2
  Sum1/1 -> Multiport Switch/2
  Sum/1 -> Sum1/1
  win/1 -> Gain3/1
  vin/1 -> Sum/1
  beta1/1 -> Sum/2
  f(vno)/1 -> Product/2
  beta4/1 -> Product/1
  Product/1 -> Multiport Switch/5
  v/1 -> Product1/1, beta4/1, beta3/1, beta1/1
  beta3/1 -> Multiport Switch/4
  Multiport Switch/1 -> vgain/1
  q/1 -> Multiport Switch/1

== system heart_model/Heart Model/VENTRICLE/CS_LV (28)/Subsystem3/Subsystem2 ==
  I_st : Inport
  q : Inport  Port=2
  vgain : Inport  Port=3
  vin : Inport  Port=4
  Compare To Constant : simulink/Logic and Bit Operations/Compare To Constant  relop===  const=2  OutDataTypeStr=uint8
  Sum : Sum  Inputs=|++
  Sum1 : Sum  Inputs=|++
  Switch : Switch  Criteria=u2 ~= 0
  vint : Outport
  wires:
  Sum1/1 -> Switch/1
  Sum/1 -> Sum1/2
  vin/1 -> Sum/2
  I_st/1 -> Sum/1
  vgain/1 -> Sum1/1, Switch/3
  Switch/1 -> vint/1
  q/1 -> Compare To Constant/1
  Compare To Constant/1 -> Switch/2

== system heart_model/Heart Model/VENTRICLE/His_d (7)/Subsystem3/Subsystem ==
  q : Inport
  v : Inport  Port=2
  f(vno) : Inport  Port=3
  vin : Inport  Port=4
  win : Inport  Port=5
  Gain3 : Gain  Gain=-1
  Multiport Switch : MultiPortSwitch  Inputs=4
  Product : Product  RndMeth=Zero
  Product1 : Product  RndMeth=Zero
  Sum : Sum  Inputs=|++
  Sum1 : Sum  Inputs=|++
  beta1 : Gain  Gain=beta1(7)
  beta3 : Gain  Gain=beta3(7)
  beta4 : Gain  Gain=beta4(7)
  vgain : Outport
  wires:
  Gain3/1 -> Product1/2
  Product1/1 -> Multiport Switch/3, Sum1/2
  Sum1/1 -> Multiport Switch/2
  Sum/1 -> Sum1/1
  win/1 -> Gain3/1
  vin/1 -> Sum/1
  beta1/1 -> Sum/2
  f(vno)/1 -> Product/2
  beta4/1 -> Product/1
  Product/1 -> Multiport Switch/5
  v/1 -> Product1/1, beta4/1, beta3/1, beta1/1
  beta3/1 -> Multiport Switch/4
  Multiport Switch/1 -> vgain/1
  q/1 -> Multiport Switch/1

== system heart_model/Heart Model/VENTRICLE/His_d (7)/Subsystem3/Subsystem2 ==
  I_st : Inport
  q : Inport  Port=2
  vgain : Inport  Port=3
  vin : Inport  Port=4
  Compare To Constant : simulink/Logic and Bit Operations/Compare To Constant  relop===  const=2  OutDataTypeStr=uint8
  Sum : Sum  Inputs=|++
  Sum1 : Sum  Inputs=|++
  Switch : Switch  Criteria=u2 ~= 0
  vint : Outport
  wires:
  Sum1/1 -> Switch/1
  Sum/1 -> Sum1/2
  vin/1 -> Sum/2
  I_st/1 -> Sum/1
  vgain/1 -> Sum1/1, Switch/3
  Switch/1 -> vint/1
  q/1 -> Compare To Constant/1
  Compare To Constant/1 -> Switch/2

== system heart_model/Heart Model/VENTRICLE/His_m (6)/Subsystem3/Subsystem ==
  q : Inport
  v : Inport  Port=2
  f(vno) : Inport  Port=3
  vin : Inport  Port=4
  win : Inport  Port=5
  Gain3 : Gain  Gain=-1
  Multiport Switch : MultiPortSwitch  Inputs=4
  Product : Product  RndMeth=Zero
  Product1 : Product  RndMeth=Zero
  Sum : Sum  Inputs=|++
  Sum1 : Sum  Inputs=|++
  beta1 : Gain  Gain=beta1(6)
  beta3 : Gain  Gain=beta3(6)
  beta4 : Gain  Gain=beta4(6)
  vgain : Outport
  wires:
  Gain3/1 -> Product1/2
  Product1/1 -> Multiport Switch/3, Sum1/2
  Sum1/1 -> Multiport Switch/2
  Sum/1 -> Sum1/1
  win/1 -> Gain3/1
  vin/1 -> Sum/1
  beta1/1 -> Sum/2
  f(vno)/1 -> Product/2
  beta4/1 -> Product/1
  Product/1 -> Multiport Switch/5
  v/1 -> Product1/1, beta4/1, beta3/1, beta1/1
  beta3/1 -> Multiport Switch/4
  Multiport Switch/1 -> vgain/1
  q/1 -> Multiport Switch/1

== system heart_model/Heart Model/VENTRICLE/His_m (6)/Subsystem3/Subsystem2 ==
  I_st : Inport
  q : Inport  Port=2
  vgain : Inport  Port=3
  vin : Inport  Port=4
  Compare To Constant : simulink/Logic and Bit Operations/Compare To Constant  relop===  const=2  OutDataTypeStr=uint8
  Sum : Sum  Inputs=|++
  Sum1 : Sum  Inputs=|++
  Switch : Switch  Criteria=u2 ~= 0
  vint : Outport
  wires:
  Sum1/1 -> Switch/1
  Sum/1 -> Sum1/2
  vin/1 -> Sum/2
  I_st/1 -> Sum/1
  vgain/1 -> Sum1/1, Switch/3
  Switch/1 -> vint/1
  q/1 -> Compare To Constant/1
  Compare To Constant/1 -> Switch/2

== system heart_model/Heart Model/VENTRICLE/His_p (5)/Subsystem3/Subsystem ==
  q : Inport
  v : Inport  Port=2
  f(vno) : Inport  Port=3
  vin : Inport  Port=4
  win : Inport  Port=5
  Gain3 : Gain  Gain=-1
  Multiport Switch : MultiPortSwitch  Inputs=4
  Product : Product  RndMeth=Zero
  Product1 : Product  RndMeth=Zero
  Sum : Sum  Inputs=|++
  Sum1 : Sum  Inputs=|++
  beta1 : Gain  Gain=beta1(5)
  beta3 : Gain  Gain=beta3(5)
  beta4 : Gain  Gain=beta4(5)
  vgain : Outport
  wires:
  Gain3/1 -> Product1/2
  Product1/1 -> Multiport Switch/3, Sum1/2
  Sum1/1 -> Multiport Switch/2
  Sum/1 -> Sum1/1
  win/1 -> Gain3/1
  vin/1 -> Sum/1
  beta1/1 -> Sum/2
  f(vno)/1 -> Product/2
  beta4/1 -> Product/1
  Product/1 -> Multiport Switch/5
  v/1 -> Product1/1, beta4/1, beta3/1, beta1/1
  beta3/1 -> Multiport Switch/4
  Multiport Switch/1 -> vgain/1
  q/1 -> Multiport Switch/1

== system heart_model/Heart Model/VENTRICLE/His_p (5)/Subsystem3/Subsystem2 ==
  I_st : Inport
  q : Inport  Port=2
  vgain : Inport  Port=3
  vin : Inport  Port=4
  Compare To Constant : simulink/Logic and Bit Operations/Compare To Constant  relop===  const=2  OutDataTypeStr=uint8
  Sum : Sum  Inputs=|++
  Sum1 : Sum  Inputs=|++
  Switch : Switch  Criteria=u2 ~= 0
  vint : Outport
  wires:
  Sum1/1 -> Switch/1
  Sum/1 -> Sum1/2
  vin/1 -> Sum/2
  I_st/1 -> Sum/1
  vgain/1 -> Sum1/1, Switch/3
  Switch/1 -> vint/1
  q/1 -> Compare To Constant/1
  Compare To Constant/1 -> Switch/2

== system heart_model/Heart Model/VENTRICLE/LBB (14)/Subsystem3/Subsystem ==
  q : Inport
  v : Inport  Port=2
  f(vno) : Inport  Port=3
  vin : Inport  Port=4
  win : Inport  Port=5
  Gain3 : Gain  Gain=-1
  Multiport Switch : MultiPortSwitch  Inputs=4
  Product : Product  RndMeth=Zero
  Product1 : Product  RndMeth=Zero
  Sum : Sum  Inputs=|++
  Sum1 : Sum  Inputs=|++
  beta1 : Gain  Gain=beta1(14)
  beta3 : Gain  Gain=beta3(14)
  beta4 : Gain  Gain=beta4(14)
  vgain : Outport
  wires:
  Gain3/1 -> Product1/2
  Product1/1 -> Multiport Switch/3, Sum1/2
  Sum1/1 -> Multiport Switch/2
  Sum/1 -> Sum1/1
  win/1 -> Gain3/1
  vin/1 -> Sum/1
  beta1/1 -> Sum/2
  f(vno)/1 -> Product/2
  beta4/1 -> Product/1
  Product/1 -> Multiport Switch/5
  v/1 -> Product1/1, beta4/1, beta3/1, beta1/1
  beta3/1 -> Multiport Switch/4
  Multiport Switch/1 -> vgain/1
  q/1 -> Multiport Switch/1

== system heart_model/Heart Model/VENTRICLE/LBB (14)/Subsystem3/Subsystem2 ==
  I_st : Inport
  q : Inport  Port=2
  vgain : Inport  Port=3
  vin : Inport  Port=4
  Compare To Constant : simulink/Logic and Bit Operations/Compare To Constant  relop===  const=2  OutDataTypeStr=uint8
  Sum : Sum  Inputs=|++
  Sum1 : Sum  Inputs=|++
  Switch : Switch  Criteria=u2 ~= 0
  vint : Outport
  wires:
  Sum1/1 -> Switch/1
  Sum/1 -> Sum1/2
  vin/1 -> Sum/2
  I_st/1 -> Sum/1
  vgain/1 -> Sum1/1, Switch/3
  Switch/1 -> vint/1
  q/1 -> Compare To Constant/1
  Compare To Constant/1 -> Switch/2

== system heart_model/Heart Model/VENTRICLE/LBB_m (13)/Subsystem3/Subsystem ==
  q : Inport
  v : Inport  Port=2
  f(vno) : Inport  Port=3
  vin : Inport  Port=4
  win : Inport  Port=5
  Gain3 : Gain  Gain=-1
  Multiport Switch : MultiPortSwitch  Inputs=4
  Product : Product  RndMeth=Zero
  Product1 : Product  RndMeth=Zero
  Sum : Sum  Inputs=|++
  Sum1 : Sum  Inputs=|++
  beta1 : Gain  Gain=beta1(13)
  beta3 : Gain  Gain=beta3(13)
  beta4 : Gain  Gain=beta4(13)
  vgain : Outport
  wires:
  Gain3/1 -> Product1/2
  Product1/1 -> Multiport Switch/3, Sum1/2
  Sum1/1 -> Multiport Switch/2
  Sum/1 -> Sum1/1
  win/1 -> Gain3/1
  vin/1 -> Sum/1
  beta1/1 -> Sum/2
  f(vno)/1 -> Product/2
  beta4/1 -> Product/1
  Product/1 -> Multiport Switch/5
  v/1 -> Product1/1, beta4/1, beta3/1, beta1/1
  beta3/1 -> Multiport Switch/4
  Multiport Switch/1 -> vgain/1
  q/1 -> Multiport Switch/1

== system heart_model/Heart Model/VENTRICLE/LBB_m (13)/Subsystem3/Subsystem2 ==
  I_st : Inport
  q : Inport  Port=2
  vgain : Inport  Port=3
  vin : Inport  Port=4
  Compare To Constant : simulink/Logic and Bit Operations/Compare To Constant  relop===  const=2  OutDataTypeStr=uint8
  Sum : Sum  Inputs=|++
  Sum1 : Sum  Inputs=|++
  Switch : Switch  Criteria=u2 ~= 0
  vint : Outport
  wires:
  Sum1/1 -> Switch/1
  Sum/1 -> Sum1/2
  vin/1 -> Sum/2
  I_st/1 -> Sum/1
  vgain/1 -> Sum1/1, Switch/3
  Switch/1 -> vint/1
  q/1 -> Compare To Constant/1
  Compare To Constant/1 -> Switch/2

== system heart_model/Heart Model/VENTRICLE/LV (20)/Subsystem3/Subsystem ==
  q : Inport
  v : Inport  Port=2
  f(vno) : Inport  Port=3
  vin : Inport  Port=4
  win : Inport  Port=5
  Gain3 : Gain  Gain=-1
  Multiport Switch : MultiPortSwitch  Inputs=4
  Product : Product  RndMeth=Zero
  Product1 : Product  RndMeth=Zero
  Sum : Sum  Inputs=|++
  Sum1 : Sum  Inputs=|++
  beta1 : Gain  Gain=beta1(20)
  beta3 : Gain  Gain=beta3(20)
  beta4 : Gain  Gain=beta4(20)
  vgain : Outport
  wires:
  Gain3/1 -> Product1/2
  Product1/1 -> Multiport Switch/3, Sum1/2
  Sum1/1 -> Multiport Switch/2
  Sum/1 -> Sum1/1
  win/1 -> Gain3/1
  vin/1 -> Sum/1
  beta1/1 -> Sum/2
  f(vno)/1 -> Product/2
  beta4/1 -> Product/1
  Product/1 -> Multiport Switch/5
  v/1 -> Product1/1, beta4/1, beta3/1, beta1/1
  beta3/1 -> Multiport Switch/4
  Multiport Switch/1 -> vgain/1
  q/1 -> Multiport Switch/1

== system heart_model/Heart Model/VENTRICLE/LV (20)/Subsystem3/Subsystem2 ==
  I_st : Inport
  q : Inport  Port=2
  vgain : Inport  Port=3
  vin : Inport  Port=4
  Compare To Constant : simulink/Logic and Bit Operations/Compare To Constant  relop===  const=2  OutDataTypeStr=uint8
  Sum : Sum  Inputs=|++
  Sum1 : Sum  Inputs=|++
  Switch : Switch  Criteria=u2 ~= 0
  vint : Outport
  wires:
  Sum1/1 -> Switch/1
  Sum/1 -> Sum1/2
  vin/1 -> Sum/2
  I_st/1 -> Sum/1
  vgain/1 -> Sum1/1, Switch/3
  Switch/1 -> vint/1
  q/1 -> Compare To Constant/1
  Compare To Constant/1 -> Switch/2

== system heart_model/Heart Model/VENTRICLE/LVA (16)/Subsystem3/Subsystem ==
  q : Inport
  v : Inport  Port=2
  f(vno) : Inport  Port=3
  vin : Inport  Port=4
  win : Inport  Port=5
  Gain3 : Gain  Gain=-1
  Multiport Switch : MultiPortSwitch  Inputs=4
  Product : Product  RndMeth=Zero
  Product1 : Product  RndMeth=Zero
  Sum : Sum  Inputs=|++
  Sum1 : Sum  Inputs=|++
  beta1 : Gain  Gain=beta1(16)
  beta3 : Gain  Gain=beta3(16)
  beta4 : Gain  Gain=beta4(16)
  vgain : Outport
  wires:
  Gain3/1 -> Product1/2
  Product1/1 -> Multiport Switch/3, Sum1/2
  Sum1/1 -> Multiport Switch/2
  Sum/1 -> Sum1/1
  win/1 -> Gain3/1
  vin/1 -> Sum/1
  beta1/1 -> Sum/2
  f(vno)/1 -> Product/2
  beta4/1 -> Product/1
  Product/1 -> Multiport Switch/5
  v/1 -> Product1/1, beta4/1, beta3/1, beta1/1
  beta3/1 -> Multiport Switch/4
  Multiport Switch/1 -> vgain/1
  q/1 -> Multiport Switch/1

== system heart_model/Heart Model/VENTRICLE/LVA (16)/Subsystem3/Subsystem2 ==
  I_st : Inport
  q : Inport  Port=2
  vgain : Inport  Port=3
  vin : Inport  Port=4
  Compare To Constant : simulink/Logic and Bit Operations/Compare To Constant  relop===  const=2  OutDataTypeStr=uint8
  Sum : Sum  Inputs=|++
  Sum1 : Sum  Inputs=|++
  Switch : Switch  Criteria=u2 ~= 0
  vint : Outport
  wires:
  Sum1/1 -> Switch/1
  Sum/1 -> Sum1/2
  vin/1 -> Sum/2
  I_st/1 -> Sum/1
  vgain/1 -> Sum1/1, Switch/3
  Switch/1 -> vint/1
  q/1 -> Compare To Constant/1
  Compare To Constant/1 -> Switch/2

== system heart_model/Heart Model/VENTRICLE/LV_m (19)/Subsystem3/Subsystem ==
  q : Inport
  v : Inport  Port=2
  f(vno) : Inport  Port=3
  vin : Inport  Port=4
  win : Inport  Port=5
  Gain3 : Gain  Gain=-1
  Multiport Switch : MultiPortSwitch  Inputs=4
  Product : Product  RndMeth=Zero
  Product1 : Product  RndMeth=Zero
  Sum : Sum  Inputs=|++
  Sum1 : Sum  Inputs=|++
  beta1 : Gain  Gain=beta1(19)
  beta3 : Gain  Gain=beta3(19)
  beta4 : Gain  Gain=beta4(19)
  vgain : Outport
  wires:
  Gain3/1 -> Product1/2
  Product1/1 -> Multiport Switch/3, Sum1/2
  Sum1/1 -> Multiport Switch/2
  Sum/1 -> Sum1/1
  win/1 -> Gain3/1
  vin/1 -> Sum/1
  beta1/1 -> Sum/2
  f(vno)/1 -> Product/2
  beta4/1 -> Product/1
  Product/1 -> Multiport Switch/5
  v/1 -> Product1/1, beta4/1, beta3/1, beta1/1
  beta3/1 -> Multiport Switch/4
  Multiport Switch/1 -> vgain/1
  q/1 -> Multiport Switch/1

== system heart_model/Heart Model/VENTRICLE/LV_m (19)/Subsystem3/Subsystem2 ==
  I_st : Inport
  q : Inport  Port=2
  vgain : Inport  Port=3
  vin : Inport  Port=4
  Compare To Constant : simulink/Logic and Bit Operations/Compare To Constant  relop===  const=2  OutDataTypeStr=uint8
  Sum : Sum  Inputs=|++
  Sum1 : Sum  Inputs=|++
  Switch : Switch  Criteria=u2 ~= 0
  vint : Outport
  wires:
  Sum1/1 -> Switch/1
  Sum/1 -> Sum1/2
  vin/1 -> Sum/2
  I_st/1 -> Sum/1
  vgain/1 -> Sum1/1, Switch/3
  Switch/1 -> vint/1
  q/1 -> Compare To Constant/1
  Compare To Constant/1 -> Switch/2

== system heart_model/Heart Model/VENTRICLE/RBB (12)/Subsystem3/Subsystem ==
  q : Inport
  v : Inport  Port=2
  f(vno) : Inport  Port=3
  vin : Inport  Port=4
  win : Inport  Port=5
  Gain3 : Gain  Gain=-1
  Multiport Switch : MultiPortSwitch  Inputs=4
  Product : Product  RndMeth=Zero
  Product1 : Product  RndMeth=Zero
  Sum : Sum  Inputs=|++
  Sum1 : Sum  Inputs=|++
  beta1 : Gain  Gain=beta1(12)
  beta3 : Gain  Gain=beta3(12)
  beta4 : Gain  Gain=beta4(12)
  vgain : Outport
  wires:
  Gain3/1 -> Product1/2
  Product1/1 -> Multiport Switch/3, Sum1/2
  Sum1/1 -> Multiport Switch/2
  Sum/1 -> Sum1/1
  win/1 -> Gain3/1
  vin/1 -> Sum/1
  beta1/1 -> Sum/2
  f(vno)/1 -> Product/2
  beta4/1 -> Product/1
  Product/1 -> Multiport Switch/5
  v/1 -> Product1/1, beta4/1, beta3/1, beta1/1
  beta3/1 -> Multiport Switch/4
  Multiport Switch/1 -> vgain/1
  q/1 -> Multiport Switch/1

== system heart_model/Heart Model/VENTRICLE/RBB (12)/Subsystem3/Subsystem2 ==
  I_st : Inport
  q : Inport  Port=2
  vgain : Inport  Port=3
  vin : Inport  Port=4
  Compare To Constant : simulink/Logic and Bit Operations/Compare To Constant  relop===  const=2  OutDataTypeStr=uint8
  Sum : Sum  Inputs=|++
  Sum1 : Sum  Inputs=|++
  Switch : Switch  Criteria=u2 ~= 0
  vint : Outport
  wires:
  Sum1/1 -> Switch/1
  Sum/1 -> Sum1/2
  vin/1 -> Sum/2
  I_st/1 -> Sum/1
  vgain/1 -> Sum1/1, Switch/3
  Switch/1 -> vint/1
  q/1 -> Compare To Constant/1
  Compare To Constant/1 -> Switch/2

== system heart_model/Heart Model/VENTRICLE/RBB_m (11)/Subsystem3/Subsystem ==
  q : Inport
  v : Inport  Port=2
  f(vno) : Inport  Port=3
  vin : Inport  Port=4
  win : Inport  Port=5
  Gain3 : Gain  Gain=-1
  Multiport Switch : MultiPortSwitch  Inputs=4
  Product : Product  RndMeth=Zero
  Product1 : Product  RndMeth=Zero
  Sum : Sum  Inputs=|++
  Sum1 : Sum  Inputs=|++
  beta1 : Gain  Gain=beta1(11)
  beta3 : Gain  Gain=beta3(11)
  beta4 : Gain  Gain=beta4(11)
  vgain : Outport
  wires:
  Gain3/1 -> Product1/2
  Product1/1 -> Multiport Switch/3, Sum1/2
  Sum1/1 -> Multiport Switch/2
  Sum/1 -> Sum1/1
  win/1 -> Gain3/1
  vin/1 -> Sum/1
  beta1/1 -> Sum/2
  f(vno)/1 -> Product/2
  beta4/1 -> Product/1
  Product/1 -> Multiport Switch/5
  v/1 -> Product1/1, beta4/1, beta3/1, beta1/1
  beta3/1 -> Multiport Switch/4
  Multiport Switch/1 -> vgain/1
  q/1 -> Multiport Switch/1

== system heart_model/Heart Model/VENTRICLE/RBB_m (11)/Subsystem3/Subsystem2 ==
  I_st : Inport
  q : Inport  Port=2
  vgain : Inport  Port=3
  vin : Inport  Port=4
  Compare To Constant : simulink/Logic and Bit Operations/Compare To Constant  relop===  const=2  OutDataTypeStr=uint8
  Sum : Sum  Inputs=|++
  Sum1 : Sum  Inputs=|++
  Switch : Switch  Criteria=u2 ~= 0
  vint : Outport
  wires:
  Sum1/1 -> Switch/1
  Sum/1 -> Sum1/2
  vin/1 -> Sum/2
  I_st/1 -> Sum/1
  vgain/1 -> Sum1/1, Switch/3
  Switch/1 -> vint/1
  q/1 -> Compare To Constant/1
  Compare To Constant/1 -> Switch/2

== system heart_model/Heart Model/VENTRICLE/RV (18)/Subsystem3/Subsystem ==
  q : Inport
  v : Inport  Port=2
  f(vno) : Inport  Port=3
  vin : Inport  Port=4
  win : Inport  Port=5
  Gain3 : Gain  Gain=-1
  Multiport Switch : MultiPortSwitch  Inputs=4
  Product : Product  RndMeth=Zero
  Product1 : Product  RndMeth=Zero
  Sum : Sum  Inputs=|++
  Sum1 : Sum  Inputs=|++
  beta1 : Gain  Gain=beta1(18)
  beta3 : Gain  Gain=beta3(18)
  beta4 : Gain  Gain=beta4(18)
  vgain : Outport
  wires:
  Gain3/1 -> Product1/2
  Product1/1 -> Multiport Switch/3, Sum1/2
  Sum1/1 -> Multiport Switch/2
  Sum/1 -> Sum1/1
  win/1 -> Gain3/1
  vin/1 -> Sum/1
  beta1/1 -> Sum/2
  f(vno)/1 -> Product/2
  beta4/1 -> Product/1
  Product/1 -> Multiport Switch/5
  v/1 -> Product1/1, beta4/1, beta3/1, beta1/1
  beta3/1 -> Multiport Switch/4
  Multiport Switch/1 -> vgain/1
  q/1 -> Multiport Switch/1

== system heart_model/Heart Model/VENTRICLE/RV (18)/Subsystem3/Subsystem2 ==
  I_st : Inport
  q : Inport  Port=2
  vgain : Inport  Port=3
  vin : Inport  Port=4
  Compare To Constant : simulink/Logic and Bit Operations/Compare To Constant  relop===  const=2  OutDataTypeStr=uint8
  Sum : Sum  Inputs=|++
  Sum1 : Sum  Inputs=|++
  Switch : Switch  Criteria=u2 ~= 0
  vint : Outport
  wires:
  Sum1/1 -> Switch/1
  Sum/1 -> Sum1/2
  vin/1 -> Sum/2
  I_st/1 -> Sum/1
  vgain/1 -> Sum1/1, Switch/3
  Switch/1 -> vint/1
  q/1 -> Compare To Constant/1
  Compare To Constant/1 -> Switch/2
